simulink model "some_testing"  (R2013a)
settings: Solver=ode45  StartTime=0.0  StopTime=30  RelTol=1e-3
values from neighbouring files (symbols this model uses):
  add_usys_d =     [tmp_wrkspc.mat]
  U_x_bounds = [-5 5]    [tmp_wrkspc.mat]
undefined symbols (not defined in the file or in its folder): ExplicitRobustMPC_obj
libraries: Robust_MPC_Library x1
settings Model: Creator=Kostas  LastModifiedBy=Kostas

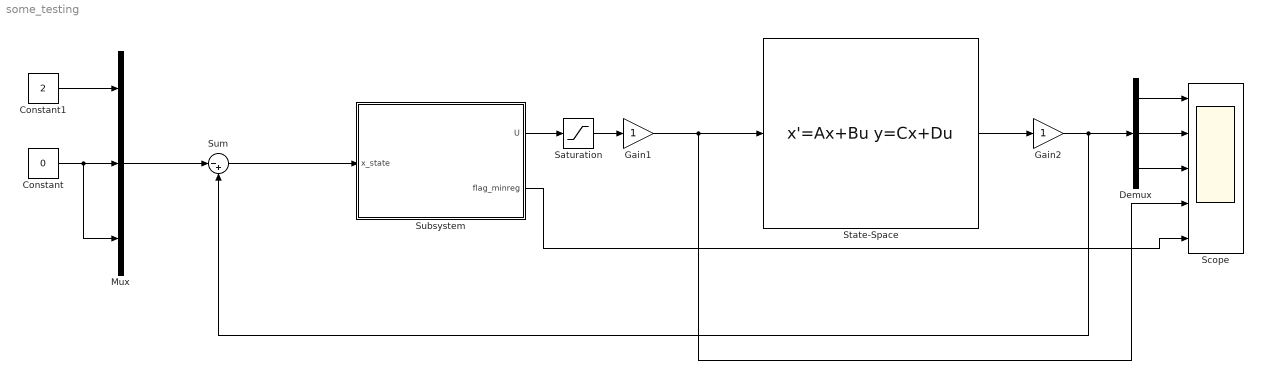
== system some_testing ==
  Constant : Constant  Value=0
  Constant1 : Constant  Value=2
  Demux : Demux  Outputs=3
  Gain1 : Gain  SampleTime=ExplicitRobustMPC_obj.Ts
  Gain2 : Gain  SampleTime=ExplicitRobustMPC_obj.Ts
  Mux : Mux  Inputs=3
  Saturation : Saturate  UpperLimit=U_x_bounds(2)  LowerLimit=U_x_bounds(1)
  Scope : Scope  NumInputPorts=5
      settings: YMin=-0.1525~0.1055~0.011~-5~-5  YMax=-0.1275~0.109~0.016~5~5
  State-Space : StateSpace  A=add_usys_d.continuous.matrices.A  B=add_usys_d.continuous.matrices.B  C=add_usys_d.continuous.matrices.C  D=add_usys_d.continuous.matrices.D  X0=[1 0 0]
  Subsystem : Subsystem
  Sum : Sum  Inputs=|-+
  wires:
  State-Space/1 -> Gain2/1
  Demux/1 -> Scope/1
  Demux/2 -> Scope/2
  Demux/3 -> Scope/3
  Subsystem/1(U) -> Saturation/1
  Saturation/1 -> Gain1/1
  Constant/1 -> Mux/3, Mux/2
  Mux/1 -> Sum/1
  Gain1/1 -> Scope/4, State-Space/1
  Constant1/1 -> Mux/1
  Gain2/1 -> Sum/2, Demux/1
  Subsystem/2(flag_minreg) -> Scope/5
  Sum/1 -> Subsystem/1(x_state)

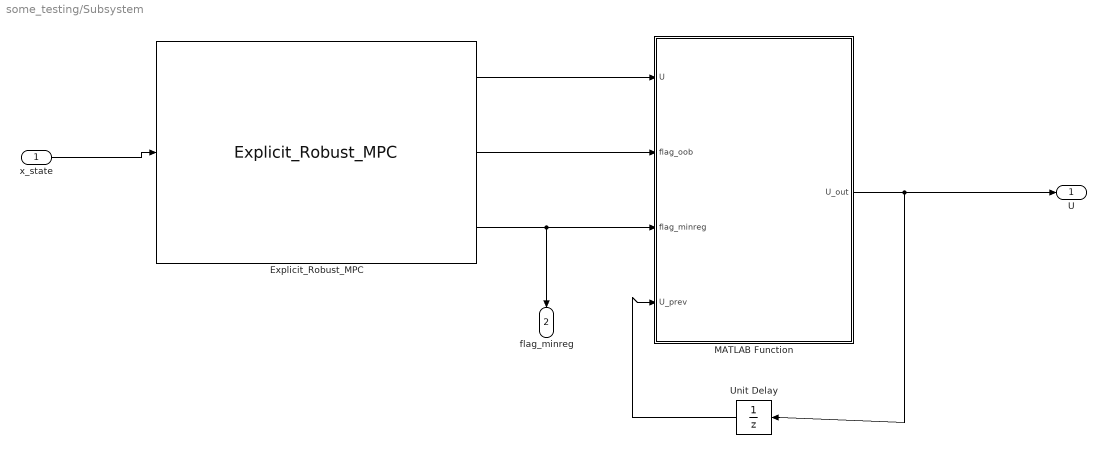
== system some_testing/Subsystem ==
  x_state : Inport
  Explicit_Robust_MPC : Robust_MPC_Library/Explicit_Robust_MPC  H=ExplicitRobustMPC_obj.H  K=ExplicitRobustMPC_obj.K  F=ExplicitRobustMPC_obj.F  G=ExplicitRobustMPC_obj.G  Nc=ExplicitRobustMPC_obj.Nc  Nx=ExplicitRobustMPC_obj.Nx  Hi_init=zeros(100,ExplicitRobustMPC_obj.Nx)  Ki_init=zeros(100,ExplicitRobustMPC_obj.Nu)
  MATLAB Function : MATLAB Function  TreatAsAtomicUnit=on
  Unit Delay : UnitDelay  SampleTime=-1
  U : Outport
  flag_minreg : Outport  Port=2
  wires:
  x_state/1 -> Explicit_Robust_MPC/1
  Explicit_Robust_MPC/1 -> MATLAB Function/1(U)
  Explicit_Robust_MPC/2 -> MATLAB Function/2(flag_oob)
  Explicit_Robust_MPC/3 -> flag_minreg/1, MATLAB Function/3(flag_minreg)
  MATLAB Function/1(U_out) -> U/1, Unit Delay/1
  Unit Delay/1 -> MATLAB Function/4(U_prev)

== matlab function some_testing/Subsystem/MATLAB Function ==
  data: U input; U_out output; flag_oob input; flag_minreg input; U_prev input
function U_out = apply_safety_rules(U,flag_oob,flag_minreg,U_prev)
%#codegen

U_out = U;

if (flag_minreg == 1)
    U_out = 0;
end

end
